simulink model "magasin"  (Simulink 6.0)
settings: Solver=ode45  SolverMode=SingleTasking  StartTime=0.0  StopTime=84.0  RelTol=1e-3
settings Model: LastModifiedBy=Seki1
settings DataIOCC: LimitDataPoints=off
settings OptimizationCC: BooleanDataType=off
settings DebuggingCC: SolverPrmCheckMsg=none
settings HardwareCC: TargetUnknown=on

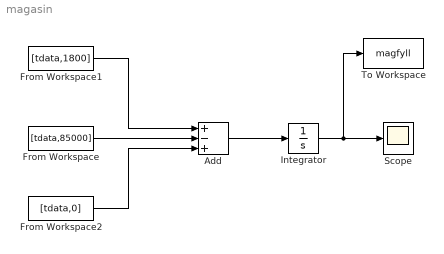
== system magasin ==
  Add : Sum  Inputs=+-+  OutScaling=2^-10
  From Workspace : FromWorkspace  VariableName=[tdata,85000]
  From Workspace1 : FromWorkspace  VariableName=[tdata,1800]
  From Workspace2 : FromWorkspace  VariableName=[tdata,0]
  Integrator : Integrator
  Scope : Scope
      settings: TickLabels=on  TimeRange=100  YMin=0  YMax=40000  DataFormat=Array
  To Workspace : ToWorkspace  VariableName=magfyll  SampleTime=-1  SaveFormat=Array
  wires:
  From Workspace1/1 -> Add/1
  From Workspace/1 -> Add/2
  From Workspace2/1 -> Add/3
  Add/1 -> Integrator/1
  Integrator/1 -> Scope/1, To Workspace/1
